simulink model "bandpass"  (R2016a)
settings: Solver=VariableStepAuto  StartTime=0.0  StopTime=5.5  RelTol=1e-3
undefined symbols (not defined in the file): fdesignblkfcn, gcbh
libraries: dspvision x4
(part 4 of 4)

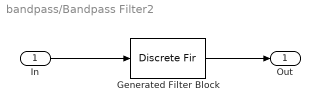
== system bandpass/Bandpass Filter2 ==
  In : Inport
  Generated Filter Block : DiscreteFir  Tag=BlockMethodSubSystem  Coefficients=[-0.00050072146804322351 3.651312600772147e-05 0.00015837852639279275 0.00036654619576597942 0.00066294831032706386 0.0010446025561711239 0.0015013355298062058 0.0020151724459947962 0.0025599887814828784 0.0031028446403869288 0.0036058217632088359 0.0040291245960319385 0.00433450900662017 0.0044894316511228756 0.0044704749819674929 0.0042669322955712309 0.003882695776323383 0.0033375214766893238 0.0026661867107773446 0.001916967875207522 0.0011475786263679556 0.00042082307951061252 -0.00020177139859217679 -0.00066560288411149241 -0.00092955571835335368 -0.00096993244117362374 -0.00078460289627773282 -0.00039333371039722786 0.00016160728667140984 0.00081963322287443956 0.0015057058550597665 0.00214082676666856 0.0026472500989640105 0.0029546020555949828 0.0030151063180480497 0.002801300689828444 0.0023160147135564239 0.0015899626006868036 0.00068186899827912535 -0.00032822782390596602 -0.0013453193584434956 -0.0022702714757163573 -0.0030096998328897318 -0.0034872720087471259 -0.0036525177442734442 -0.0034882696693712086 -0.003013631074395244 -0.0022842966730344449 -0.0013877547856772578 -0.00043559294838993012 0.00044815756609056226 0.0011397733296877395 0.0015302860783442077 0.0015379932118380166 0.0011194897313586364 0.00027614666558852327 -0.00094301002161820342 -0.0024446767383302904 -0.0040986718774789323 -0.0057513690029963082 -0.0072408662988688232 -0.008415173928891042 -0.0091487708913831518 -0.0093601066202952891 -0.0090213203401396293 -0.0081651311783551839 -0.0068853337705290715 -0.005328458377070442 -0.0036816748940217063 -0.0021533069393916702 -0.00095144041848531325 -0.00025995239949081281 -0.00021704630824168568 -0.00089643405426797324 -0.0022953894087262309 -0.0043301385051047183 -0.0068398833680354499 -0.0095997041632244276 -0.012341391300356244 -0.014780224913929803 -0.016645363281454165 -0.017710823866591726 -0.017823437413187409 -0.016924809039356833 -0.015064611776916379 -0.012403108137440725 -0.0092018957591263936 -0.0058031237193337092 -0.0025986330322102682 8.3692445053706102e-06 0.0016455294324835871 0.0020140161583015719 0.00092649468274067079 -0.0016632850574367 -0.0056432341159023992 -0.010738814525976687 -0.016526511882006923 -0.022460903076231005 -0.027916080607798262 -0.032237582790487468 -0.034799770397695821 -0.035064855918146003 -0.032636714395371559 -0.027306033617417281 -0.019080034726856768 -0.0081963508840238123 0.0048838511564608658 0.019501265236993325 0.034841915195635904 0.049994967683452893 0.064020660143298963 0.07602191871921922 0.085214345718042386 0.090988175775337382 0.092956919150096531 0.090988175775337382 0.085214345718042386 0.07602191871921922 0.064020660143298963 0.049994967683452893 0.034841915195635904 0.019501265236993325 0.0048838511564608658 -0.0081963508840238123 -0.019080034726856768 -0.027306033617417281 -0.032636714395371559 -0.035064855918146003 -0.034799770397695821 -0.032237582790487468 -0.027916080607798262 -0.022460903076231005 -0.016526511882006923 -0.010738814525976687 -0.0056432341159023992 -0.0016632850574367 0.00092649468274067079 0.0020140161583015719 0.0016455294324835871 8.3692445053706102e-06 -0.0025986330322102682 -0.0058031237193337092 -0.0092018957591263936 -0.012403108137440725 -0.015064611776916379 -0.016924809039356833 -0.017823437413187409 -0.017710823866591726 -0.016645363281454165 -0.014780224913929803 -0.012341391300356244 -0.0095997041632244276 -0.0068398833680354499 -0.0043301385051047183 -0.0022953894087262309 -0.00089643405426797324 -0.00021704630824168568 -0.00025995239949081281 -0.00095144041848531325 -0.0021533069393916702 -0.0036816748940217063 -0.005328458377070442 -0.0068853337705290715 -0.0081651311783551839 -0.0090213203401396293 -0.0093601066202952891 -0.0091487708913831518 -0.008415173928891042 -0.0072408662988688232 -0.0057513690029963082 -0.0040986718774789323 -0.0024446767383302904 -0.00094301002161820342 0.00027614666558852327 0.0011194897313586364 0.0015379932118380166 0.0015302860783442077 0.0011397733296877395 ...(+1149 chars)]  InputProcessing=Columns as channels (frame based)
  Out : Outport
  wires:
  In/1 -> Generated Filter Block/1
  Generated Filter Block/1 -> Out/1
